simulink model "decoder8to256"  (R2020a)
settings: Solver=VariableStepAuto  StartTime=0.0  StopTime=10.0  RelTol=1e-3
(part 2 of 2)

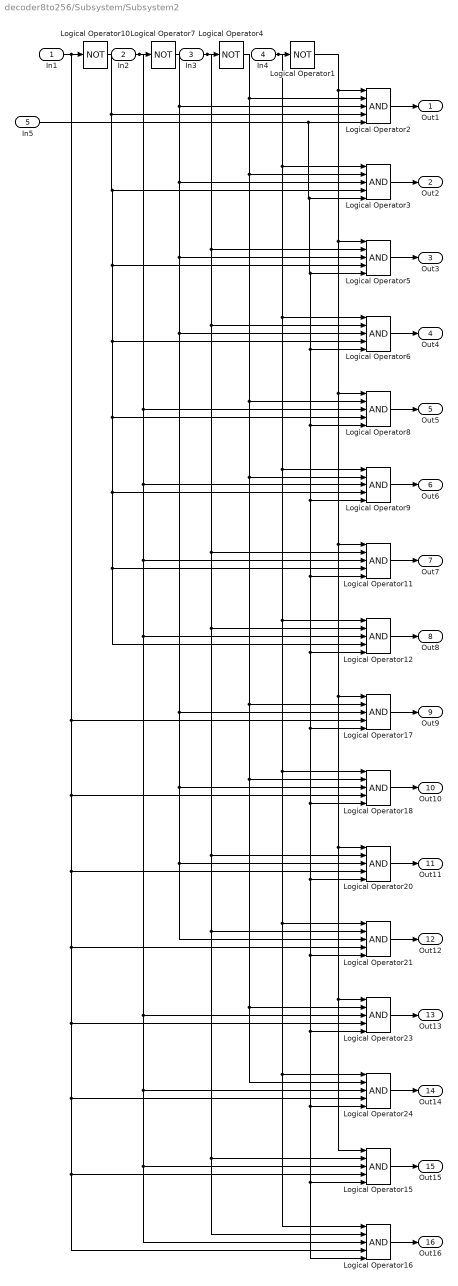
== system decoder8to256/Subsystem/Subsystem2 ==
  In1 : Inport
  In2 : Inport  Port=2
  In3 : Inport  Port=3
  In4 : Inport  Port=4
  In5 : Inport  Port=5
  Logical Operator{1,4,7,10} (4 alike) : Logic  Operator=NOT  AllPortsSameDT=off  OutDataTypeStr=boolean
  Logical Operator{2..3,5..6,8..9,11..12,15..18,20..21,23..24} (16 alike) : Logic  Inputs=5  AllPortsSameDT=off  OutDataTypeStr=boolean
  Out1 : Outport
  Out2 : Outport  Port=2
  Out3 : Outport  Port=3
  Out4 : Outport  Port=4
  Out5 : Outport  Port=5
  Out6 : Outport  Port=6
  Out7 : Outport  Port=7
  Out8 : Outport  Port=8
  Out9 : Outport  Port=9
  Out10 : Outport  Port=10
  Out11 : Outport  Port=11
  Out12 : Outport  Port=12
  Out13 : Outport  Port=13
  Out14 : Outport  Port=14
  Out15 : Outport  Port=15
  Out16 : Outport  Port=16
  wires:
  Logical Operator11/1 -> Out7/1
  Logical Operator12/1 -> Out8/1
  Logical Operator18/1 -> Out10/1
  In2/1 -> Logical Operator16/3, Logical Operator15/3, Logical Operator24/3, Logical Operator23/3, Logical Operator12/3, Logical Operator11/3, Logical Operator9/3, Logical Operator8/3, Logical Operator7/1
  In3/1 -> Logical Operator11/2, Logical Operator15/2, Logical Operator16/2, Logical Operator21/2, Logical Operator20/2, Logical Operator12/2, Logical Operator6/2, Logical Operator5/2, Logical Operator4/1
  Logical Operator24/1 -> Out14/1
  In4/1 -> Logical Operator16/1, Logical Operator24/1, Logical Operator21/1, Logical Operator18/1, Logical Operator12/1, Logical Operator9/1, Logical Operator6/1, Logical Operator3/1, Logical Operator1/1
  Logical Operator10/1 -> Logical Operator12/4, Logical Operator11/4, Logical Operator9/4, Logical Operator8/4, Logical Operator6/4, Logical Operator5/4, Logical Operator3/4, Logical Operator2/4
  Logical Operator9/1 -> Out6/1
  In5/1 -> Logical Operator16/5, Logical Operator15/5, Logical Operator24/5, Logical Operator23/5, Logical Operator21/5, Logical Operator20/5, Logical Operator18/5, Logical Operator17/5, Logical Operator12/5, Logical Operator11/5, Logical Operator9/5, Logical Operator8/5, Logical Operator6/5, Logical Operator5/5, Logical Operator3/5, Logical Operator2/5
  Logical Operator5/1 -> Out3/1
  Logical Operator1/1 -> Logical Operator15/1, Logical Operator23/1, Logical Operator20/1, Logical Operator17/1, Logical Operator11/1, Logical Operator8/1, Logical Operator5/1, Logical Operator2/1
  Logical Operator2/1 -> Out1/1
  Logical Operator21/1 -> Out12/1
  Logical Operator8/1 -> Out5/1
  Logical Operator7/1 -> Logical Operator21/3, Logical Operator20/3, Logical Operator18/3, Logical Operator17/3, Logical Operator6/3, Logical Operator5/3, Logical Operator3/3, Logical Operator2/3
  Logical Operator16/1 -> Out16/1
  Logical Operator15/1 -> Out15/1
  In1/1 -> Logical Operator17/4, Logical Operator18/4, Logical Operator20/4, Logical Operator21/4, Logical Operator23/4, Logical Operator24/4, Logical Operator15/4, Logical Operator16/4, Logical Operator10/1
  Logical Operator3/1 -> Out2/1
  Logical Operator20/1 -> Out11/1
  Logical Operator6/1 -> Out4/1
  Logical Operator23/1 -> Out13/1
  Logical Operator4/1 -> Logical Operator24/2, Logical Operator23/2, Logical Operator18/2, Logical Operator17/2, Logical Operator9/2, Logical Operator8/2, Logical Operator3/2, Logical Operator2/2
  Logical Operator17/1 -> Out9/1

== system decoder8to256/Subsystem/Subsystem3 ==
  In1 : Inport
  In2 : Inport  Port=2
  In3 : Inport  Port=3
  In4 : Inport  Port=4
  In5 : Inport  Port=5
  Logical Operator{1,4,7,10} (4 alike) : Logic  Operator=NOT  AllPortsSameDT=off  OutDataTypeStr=boolean
  Logical Operator{2..3,5..6,8..9,11..12,15..18,20..21,23..24} (16 alike) : Logic  Inputs=5  AllPortsSameDT=off  OutDataTypeStr=boolean
  Out1 : Outport
  Out2 : Outport  Port=2
  Out3 : Outport  Port=3
  Out4 : Outport  Port=4
  Out5 : Outport  Port=5
  Out6 : Outport  Port=6
  Out7 : Outport  Port=7
  Out8 : Outport  Port=8
  Out9 : Outport  Port=9
  Out10 : Outport  Port=10
  Out11 : Outport  Port=11
  Out12 : Outport  Port=12
  Out13 : Outport  Port=13
  Out14 : Outport  Port=14
  Out15 : Outport  Port=15
  Out16 : Outport  Port=16
  wires:
  Logical Operator11/1 -> Out7/1
  Logical Operator12/1 -> Out8/1
  Logical Operator18/1 -> Out10/1
  In2/1 -> Logical Operator16/3, Logical Operator15/3, Logical Operator24/3, Logical Operator23/3, Logical Operator12/3, Logical Operator11/3, Logical Operator9/3, Logical Operator8/3, Logical Operator7/1
  In3/1 -> Logical Operator11/2, Logical Operator15/2, Logical Operator16/2, Logical Operator21/2, Logical Operator20/2, Logical Operator12/2, Logical Operator6/2, Logical Operator5/2, Logical Operator4/1
  Logical Operator24/1 -> Out14/1
  In4/1 -> Logical Operator16/1, Logical Operator24/1, Logical Operator21/1, Logical Operator18/1, Logical Operator12/1, Logical Operator9/1, Logical Operator6/1, Logical Operator3/1, Logical Operator1/1
  Logical Operator10/1 -> Logical Operator12/4, Logical Operator11/4, Logical Operator9/4, Logical Operator8/4, Logical Operator6/4, Logical Operator5/4, Logical Operator3/4, Logical Operator2/4
  Logical Operator9/1 -> Out6/1
  In5/1 -> Logical Operator16/5, Logical Operator15/5, Logical Operator24/5, Logical Operator23/5, Logical Operator21/5, Logical Operator20/5, Logical Operator18/5, Logical Operator17/5, Logical Operator12/5, Logical Operator11/5, Logical Operator9/5, Logical Operator8/5, Logical Operator6/5, Logical Operator5/5, Logical Operator3/5, Logical Operator2/5
  Logical Operator5/1 -> Out3/1
  Logical Operator1/1 -> Logical Operator15/1, Logical Operator23/1, Logical Operator20/1, Logical Operator17/1, Logical Operator11/1, Logical Operator8/1, Logical Operator5/1, Logical Operator2/1
  Logical Operator2/1 -> Out1/1
  Logical Operator21/1 -> Out12/1
  Logical Operator8/1 -> Out5/1
  Logical Operator7/1 -> Logical Operator21/3, Logical Operator20/3, Logical Operator18/3, Logical Operator17/3, Logical Operator6/3, Logical Operator5/3, Logical Operator3/3, Logical Operator2/3
  Logical Operator16/1 -> Out16/1
  Logical Operator15/1 -> Out15/1
  In1/1 -> Logical Operator17/4, Logical Operator18/4, Logical Operator20/4, Logical Operator21/4, Logical Operator23/4, Logical Operator24/4, Logical Operator15/4, Logical Operator16/4, Logical Operator10/1
  Logical Operator3/1 -> Out2/1
  Logical Operator20/1 -> Out11/1
  Logical Operator6/1 -> Out4/1
  Logical Operator23/1 -> Out13/1
  Logical Operator4/1 -> Logical Operator24/2, Logical Operator23/2, Logical Operator18/2, Logical Operator17/2, Logical Operator9/2, Logical Operator8/2, Logical Operator3/2, Logical Operator2/2
  Logical Operator17/1 -> Out9/1

== system decoder8to256/Subsystem/Subsystem4 ==
  In1 : Inport
  In2 : Inport  Port=2
  In3 : Inport  Port=3
  In4 : Inport  Port=4
  In5 : Inport  Port=5
  Logical Operator{1,4,7,10} (4 alike) : Logic  Operator=NOT  AllPortsSameDT=off  OutDataTypeStr=boolean
  Logical Operator{2..3,5..6,8..9,11..12,15..18,20..21,23..24} (16 alike) : Logic  Inputs=5  AllPortsSameDT=off  OutDataTypeStr=boolean
  Out1 : Outport
  Out2 : Outport  Port=2
  Out3 : Outport  Port=3
  Out4 : Outport  Port=4
  Out5 : Outport  Port=5
  Out6 : Outport  Port=6
  Out7 : Outport  Port=7
  Out8 : Outport  Port=8
  Out9 : Outport  Port=9
  Out10 : Outport  Port=10
  Out11 : Outport  Port=11
  Out12 : Outport  Port=12
  Out13 : Outport  Port=13
  Out14 : Outport  Port=14
  Out15 : Outport  Port=15
  Out16 : Outport  Port=16
  wires:
  Logical Operator11/1 -> Out7/1
  Logical Operator12/1 -> Out8/1
  Logical Operator18/1 -> Out10/1
  In2/1 -> Logical Operator16/3, Logical Operator15/3, Logical Operator24/3, Logical Operator23/3, Logical Operator12/3, Logical Operator11/3, Logical Operator9/3, Logical Operator8/3, Logical Operator7/1
  In3/1 -> Logical Operator11/2, Logical Operator15/2, Logical Operator16/2, Logical Operator21/2, Logical Operator20/2, Logical Operator12/2, Logical Operator6/2, Logical Operator5/2, Logical Operator4/1
  Logical Operator24/1 -> Out14/1
  In4/1 -> Logical Operator16/1, Logical Operator24/1, Logical Operator21/1, Logical Operator18/1, Logical Operator12/1, Logical Operator9/1, Logical Operator6/1, Logical Operator3/1, Logical Operator1/1
  Logical Operator10/1 -> Logical Operator12/4, Logical Operator11/4, Logical Operator9/4, Logical Operator8/4, Logical Operator6/4, Logical Operator5/4, Logical Operator3/4, Logical Operator2/4
  Logical Operator9/1 -> Out6/1
  In5/1 -> Logical Operator16/5, Logical Operator15/5, Logical Operator24/5, Logical Operator23/5, Logical Operator21/5, Logical Operator20/5, Logical Operator18/5, Logical Operator17/5, Logical Operator12/5, Logical Operator11/5, Logical Operator9/5, Logical Operator8/5, Logical Operator6/5, Logical Operator5/5, Logical Operator3/5, Logical Operator2/5
  Logical Operator5/1 -> Out3/1
  Logical Operator1/1 -> Logical Operator15/1, Logical Operator23/1, Logical Operator20/1, Logical Operator17/1, Logical Operator11/1, Logical Operator8/1, Logical Operator5/1, Logical Operator2/1
  Logical Operator2/1 -> Out1/1
  Logical Operator21/1 -> Out12/1
  Logical Operator8/1 -> Out5/1
  Logical Operator7/1 -> Logical Operator21/3, Logical Operator20/3, Logical Operator18/3, Logical Operator17/3, Logical Operator6/3, Logical Operator5/3, Logical Operator3/3, Logical Operator2/3
  Logical Operator16/1 -> Out16/1
  Logical Operator15/1 -> Out15/1
  In1/1 -> Logical Operator17/4, Logical Operator18/4, Logical Operator20/4, Logical Operator21/4, Logical Operator23/4, Logical Operator24/4, Logical Operator15/4, Logical Operator16/4, Logical Operator10/1
  Logical Operator3/1 -> Out2/1
  Logical Operator20/1 -> Out11/1
  Logical Operator6/1 -> Out4/1
  Logical Operator23/1 -> Out13/1
  Logical Operator4/1 -> Logical Operator24/2, Logical Operator23/2, Logical Operator18/2, Logical Operator17/2, Logical Operator9/2, Logical Operator8/2, Logical Operator3/2, Logical Operator2/2
  Logical Operator17/1 -> Out9/1

== system decoder8to256/Subsystem/Subsystem5 ==
  In1 : Inport
  In2 : Inport  Port=2
  In3 : Inport  Port=3
  In4 : Inport  Port=4
  In5 : Inport  Port=5
  Logical Operator{1,4,7,10} (4 alike) : Logic  Operator=NOT  AllPortsSameDT=off  OutDataTypeStr=boolean
  Logical Operator{2..3,5..6,8..9,11..12,15..18,20..21,23..24} (16 alike) : Logic  Inputs=5  AllPortsSameDT=off  OutDataTypeStr=boolean
  Out1 : Outport
  Out2 : Outport  Port=2
  Out3 : Outport  Port=3
  Out4 : Outport  Port=4
  Out5 : Outport  Port=5
  Out6 : Outport  Port=6
  Out7 : Outport  Port=7
  Out8 : Outport  Port=8
  Out9 : Outport  Port=9
  Out10 : Outport  Port=10
  Out11 : Outport  Port=11
  Out12 : Outport  Port=12
  Out13 : Outport  Port=13
  Out14 : Outport  Port=14
  Out15 : Outport  Port=15
  Out16 : Outport  Port=16
  wires:
  Logical Operator11/1 -> Out7/1
  Logical Operator12/1 -> Out8/1
  Logical Operator18/1 -> Out10/1
  In2/1 -> Logical Operator16/3, Logical Operator15/3, Logical Operator24/3, Logical Operator23/3, Logical Operator12/3, Logical Operator11/3, Logical Operator9/3, Logical Operator8/3, Logical Operator7/1
  In3/1 -> Logical Operator11/2, Logical Operator15/2, Logical Operator16/2, Logical Operator21/2, Logical Operator20/2, Logical Operator12/2, Logical Operator6/2, Logical Operator5/2, Logical Operator4/1
  Logical Operator24/1 -> Out14/1
  In4/1 -> Logical Operator16/1, Logical Operator24/1, Logical Operator21/1, Logical Operator18/1, Logical Operator12/1, Logical Operator9/1, Logical Operator6/1, Logical Operator3/1, Logical Operator1/1
  Logical Operator10/1 -> Logical Operator12/4, Logical Operator11/4, Logical Operator9/4, Logical Operator8/4, Logical Operator6/4, Logical Operator5/4, Logical Operator3/4, Logical Operator2/4
  Logical Operator9/1 -> Out6/1
  In5/1 -> Logical Operator16/5, Logical Operator15/5, Logical Operator24/5, Logical Operator23/5, Logical Operator21/5, Logical Operator20/5, Logical Operator18/5, Logical Operator17/5, Logical Operator12/5, Logical Operator11/5, Logical Operator9/5, Logical Operator8/5, Logical Operator6/5, Logical Operator5/5, Logical Operator3/5, Logical Operator2/5
  Logical Operator5/1 -> Out3/1
  Logical Operator1/1 -> Logical Operator15/1, Logical Operator23/1, Logical Operator20/1, Logical Operator17/1, Logical Operator11/1, Logical Operator8/1, Logical Operator5/1, Logical Operator2/1
  Logical Operator2/1 -> Out1/1
  Logical Operator21/1 -> Out12/1
  Logical Operator8/1 -> Out5/1
  Logical Operator7/1 -> Logical Operator21/3, Logical Operator20/3, Logical Operator18/3, Logical Operator17/3, Logical Operator6/3, Logical Operator5/3, Logical Operator3/3, Logical Operator2/3
  Logical Operator16/1 -> Out16/1
  Logical Operator15/1 -> Out15/1
  In1/1 -> Logical Operator17/4, Logical Operator18/4, Logical Operator20/4, Logical Operator21/4, Logical Operator23/4, Logical Operator24/4, Logical Operator15/4, Logical Operator16/4, Logical Operator10/1
  Logical Operator3/1 -> Out2/1
  Logical Operator20/1 -> Out11/1
  Logical Operator6/1 -> Out4/1
  Logical Operator23/1 -> Out13/1
  Logical Operator4/1 -> Logical Operator24/2, Logical Operator23/2, Logical Operator18/2, Logical Operator17/2, Logical Operator9/2, Logical Operator8/2, Logical Operator3/2, Logical Operator2/2
  Logical Operator17/1 -> Out9/1

== system decoder8to256/Subsystem/Subsystem6 ==
  In1 : Inport
  In2 : Inport  Port=2
  In3 : Inport  Port=3
  In4 : Inport  Port=4
  In5 : Inport  Port=5
  Logical Operator{1,4,7,10} (4 alike) : Logic  Operator=NOT  AllPortsSameDT=off  OutDataTypeStr=boolean
  Logical Operator{2..3,5..6,8..9,11..12,15..18,20..21,23..24} (16 alike) : Logic  Inputs=5  AllPortsSameDT=off  OutDataTypeStr=boolean
  Out1 : Outport
  Out2 : Outport  Port=2
  Out3 : Outport  Port=3
  Out4 : Outport  Port=4
  Out5 : Outport  Port=5
  Out6 : Outport  Port=6
  Out7 : Outport  Port=7
  Out8 : Outport  Port=8
  Out9 : Outport  Port=9
  Out10 : Outport  Port=10
  Out11 : Outport  Port=11
  Out12 : Outport  Port=12
  Out13 : Outport  Port=13
  Out14 : Outport  Port=14
  Out15 : Outport  Port=15
  Out16 : Outport  Port=16
  wires:
  Logical Operator11/1 -> Out7/1
  Logical Operator12/1 -> Out8/1
  Logical Operator18/1 -> Out10/1
  In2/1 -> Logical Operator16/3, Logical Operator15/3, Logical Operator24/3, Logical Operator23/3, Logical Operator12/3, Logical Operator11/3, Logical Operator9/3, Logical Operator8/3, Logical Operator7/1
  In3/1 -> Logical Operator11/2, Logical Operator15/2, Logical Operator16/2, Logical Operator21/2, Logical Operator20/2, Logical Operator12/2, Logical Operator6/2, Logical Operator5/2, Logical Operator4/1
  Logical Operator24/1 -> Out14/1
  In4/1 -> Logical Operator16/1, Logical Operator24/1, Logical Operator21/1, Logical Operator18/1, Logical Operator12/1, Logical Operator9/1, Logical Operator6/1, Logical Operator3/1, Logical Operator1/1
  Logical Operator10/1 -> Logical Operator12/4, Logical Operator11/4, Logical Operator9/4, Logical Operator8/4, Logical Operator6/4, Logical Operator5/4, Logical Operator3/4, Logical Operator2/4
  Logical Operator9/1 -> Out6/1
  In5/1 -> Logical Operator16/5, Logical Operator15/5, Logical Operator24/5, Logical Operator23/5, Logical Operator21/5, Logical Operator20/5, Logical Operator18/5, Logical Operator17/5, Logical Operator12/5, Logical Operator11/5, Logical Operator9/5, Logical Operator8/5, Logical Operator6/5, Logical Operator5/5, Logical Operator3/5, Logical Operator2/5
  Logical Operator5/1 -> Out3/1
  Logical Operator1/1 -> Logical Operator15/1, Logical Operator23/1, Logical Operator20/1, Logical Operator17/1, Logical Operator11/1, Logical Operator8/1, Logical Operator5/1, Logical Operator2/1
  Logical Operator2/1 -> Out1/1
  Logical Operator21/1 -> Out12/1
  Logical Operator8/1 -> Out5/1
  Logical Operator7/1 -> Logical Operator21/3, Logical Operator20/3, Logical Operator18/3, Logical Operator17/3, Logical Operator6/3, Logical Operator5/3, Logical Operator3/3, Logical Operator2/3
  Logical Operator16/1 -> Out16/1
  Logical Operator15/1 -> Out15/1
  In1/1 -> Logical Operator17/4, Logical Operator18/4, Logical Operator20/4, Logical Operator21/4, Logical Operator23/4, Logical Operator24/4, Logical Operator15/4, Logical Operator16/4, Logical Operator10/1
  Logical Operator3/1 -> Out2/1
  Logical Operator20/1 -> Out11/1
  Logical Operator6/1 -> Out4/1
  Logical Operator23/1 -> Out13/1
  Logical Operator4/1 -> Logical Operator24/2, Logical Operator23/2, Logical Operator18/2, Logical Operator17/2, Logical Operator9/2, Logical Operator8/2, Logical Operator3/2, Logical Operator2/2
  Logical Operator17/1 -> Out9/1

== system decoder8to256/Subsystem/Subsystem7 ==
  In1 : Inport
  In2 : Inport  Port=2
  In3 : Inport  Port=3
  In4 : Inport  Port=4
  In5 : Inport  Port=5
  Logical Operator{1,4,7,10} (4 alike) : Logic  Operator=NOT  AllPortsSameDT=off  OutDataTypeStr=boolean
  Logical Operator{2..3,5..6,8..9,11..12,15..18,20..21,23..24} (16 alike) : Logic  Inputs=5  AllPortsSameDT=off  OutDataTypeStr=boolean
  Out1 : Outport
  Out2 : Outport  Port=2
  Out3 : Outport  Port=3
  Out4 : Outport  Port=4
  Out5 : Outport  Port=5
  Out6 : Outport  Port=6
  Out7 : Outport  Port=7
  Out8 : Outport  Port=8
  Out9 : Outport  Port=9
  Out10 : Outport  Port=10
  Out11 : Outport  Port=11
  Out12 : Outport  Port=12
  Out13 : Outport  Port=13
  Out14 : Outport  Port=14
  Out15 : Outport  Port=15
  Out16 : Outport  Port=16
  wires:
  Logical Operator11/1 -> Out7/1
  Logical Operator12/1 -> Out8/1
  Logical Operator18/1 -> Out10/1
  In2/1 -> Logical Operator16/3, Logical Operator15/3, Logical Operator24/3, Logical Operator23/3, Logical Operator12/3, Logical Operator11/3, Logical Operator9/3, Logical Operator8/3, Logical Operator7/1
  In3/1 -> Logical Operator11/2, Logical Operator15/2, Logical Operator16/2, Logical Operator21/2, Logical Operator20/2, Logical Operator12/2, Logical Operator6/2, Logical Operator5/2, Logical Operator4/1
  Logical Operator24/1 -> Out14/1
  In4/1 -> Logical Operator16/1, Logical Operator24/1, Logical Operator21/1, Logical Operator18/1, Logical Operator12/1, Logical Operator9/1, Logical Operator6/1, Logical Operator3/1, Logical Operator1/1
  Logical Operator10/1 -> Logical Operator12/4, Logical Operator11/4, Logical Operator9/4, Logical Operator8/4, Logical Operator6/4, Logical Operator5/4, Logical Operator3/4, Logical Operator2/4
  Logical Operator9/1 -> Out6/1
  In5/1 -> Logical Operator16/5, Logical Operator15/5, Logical Operator24/5, Logical Operator23/5, Logical Operator21/5, Logical Operator20/5, Logical Operator18/5, Logical Operator17/5, Logical Operator12/5, Logical Operator11/5, Logical Operator9/5, Logical Operator8/5, Logical Operator6/5, Logical Operator5/5, Logical Operator3/5, Logical Operator2/5
  Logical Operator5/1 -> Out3/1
  Logical Operator1/1 -> Logical Operator15/1, Logical Operator23/1, Logical Operator20/1, Logical Operator17/1, Logical Operator11/1, Logical Operator8/1, Logical Operator5/1, Logical Operator2/1
  Logical Operator2/1 -> Out1/1
  Logical Operator21/1 -> Out12/1
  Logical Operator8/1 -> Out5/1
  Logical Operator7/1 -> Logical Operator21/3, Logical Operator20/3, Logical Operator18/3, Logical Operator17/3, Logical Operator6/3, Logical Operator5/3, Logical Operator3/3, Logical Operator2/3
  Logical Operator16/1 -> Out16/1
  Logical Operator15/1 -> Out15/1
  In1/1 -> Logical Operator17/4, Logical Operator18/4, Logical Operator20/4, Logical Operator21/4, Logical Operator23/4, Logical Operator24/4, Logical Operator15/4, Logical Operator16/4, Logical Operator10/1
  Logical Operator3/1 -> Out2/1
  Logical Operator20/1 -> Out11/1
  Logical Operator6/1 -> Out4/1
  Logical Operator23/1 -> Out13/1
  Logical Operator4/1 -> Logical Operator24/2, Logical Operator23/2, Logical Operator18/2, Logical Operator17/2, Logical Operator9/2, Logical Operator8/2, Logical Operator3/2, Logical Operator2/2
  Logical Operator17/1 -> Out9/1

== system decoder8to256/Subsystem/Subsystem8 ==
  In1 : Inport
  In2 : Inport  Port=2
  In3 : Inport  Port=3
  In4 : Inport  Port=4
  In5 : Inport  Port=5
  Logical Operator{1,4,7,10} (4 alike) : Logic  Operator=NOT  AllPortsSameDT=off  OutDataTypeStr=boolean
  Logical Operator{2..3,5..6,8..9,11..12,15..18,20..21,23..24} (16 alike) : Logic  Inputs=5  AllPortsSameDT=off  OutDataTypeStr=boolean
  Out1 : Outport
  Out2 : Outport  Port=2
  Out3 : Outport  Port=3
  Out4 : Outport  Port=4
  Out5 : Outport  Port=5
  Out6 : Outport  Port=6
  Out7 : Outport  Port=7
  Out8 : Outport  Port=8
  Out9 : Outport  Port=9
  Out10 : Outport  Port=10
  Out11 : Outport  Port=11
  Out12 : Outport  Port=12
  Out13 : Outport  Port=13
  Out14 : Outport  Port=14
  Out15 : Outport  Port=15
  Out16 : Outport  Port=16
  wires:
  Logical Operator11/1 -> Out7/1
  Logical Operator12/1 -> Out8/1
  Logical Operator18/1 -> Out10/1
  In2/1 -> Logical Operator16/3, Logical Operator15/3, Logical Operator24/3, Logical Operator23/3, Logical Operator12/3, Logical Operator11/3, Logical Operator9/3, Logical Operator8/3, Logical Operator7/1
  In3/1 -> Logical Operator11/2, Logical Operator15/2, Logical Operator16/2, Logical Operator21/2, Logical Operator20/2, Logical Operator12/2, Logical Operator6/2, Logical Operator5/2, Logical Operator4/1
  Logical Operator24/1 -> Out14/1
  In4/1 -> Logical Operator16/1, Logical Operator24/1, Logical Operator21/1, Logical Operator18/1, Logical Operator12/1, Logical Operator9/1, Logical Operator6/1, Logical Operator3/1, Logical Operator1/1
  Logical Operator10/1 -> Logical Operator12/4, Logical Operator11/4, Logical Operator9/4, Logical Operator8/4, Logical Operator6/4, Logical Operator5/4, Logical Operator3/4, Logical Operator2/4
  Logical Operator9/1 -> Out6/1
  In5/1 -> Logical Operator16/5, Logical Operator15/5, Logical Operator24/5, Logical Operator23/5, Logical Operator21/5, Logical Operator20/5, Logical Operator18/5, Logical Operator17/5, Logical Operator12/5, Logical Operator11/5, Logical Operator9/5, Logical Operator8/5, Logical Operator6/5, Logical Operator5/5, Logical Operator3/5, Logical Operator2/5
  Logical Operator5/1 -> Out3/1
  Logical Operator1/1 -> Logical Operator15/1, Logical Operator23/1, Logical Operator20/1, Logical Operator17/1, Logical Operator11/1, Logical Operator8/1, Logical Operator5/1, Logical Operator2/1
  Logical Operator2/1 -> Out1/1
  Logical Operator21/1 -> Out12/1
  Logical Operator8/1 -> Out5/1
  Logical Operator7/1 -> Logical Operator21/3, Logical Operator20/3, Logical Operator18/3, Logical Operator17/3, Logical Operator6/3, Logical Operator5/3, Logical Operator3/3, Logical Operator2/3
  Logical Operator16/1 -> Out16/1
  Logical Operator15/1 -> Out15/1
  In1/1 -> Logical Operator17/4, Logical Operator18/4, Logical Operator20/4, Logical Operator21/4, Logical Operator23/4, Logical Operator24/4, Logical Operator15/4, Logical Operator16/4, Logical Operator10/1
  Logical Operator3/1 -> Out2/1
  Logical Operator20/1 -> Out11/1
  Logical Operator6/1 -> Out4/1
  Logical Operator23/1 -> Out13/1
  Logical Operator4/1 -> Logical Operator24/2, Logical Operator23/2, Logical Operator18/2, Logical Operator17/2, Logical Operator9/2, Logical Operator8/2, Logical Operator3/2, Logical Operator2/2
  Logical Operator17/1 -> Out9/1

== system decoder8to256/Subsystem/Subsystem9 ==
  In1 : Inport
  In2 : Inport  Port=2
  In3 : Inport  Port=3
  In4 : Inport  Port=4
  In5 : Inport  Port=5
  Logical Operator{1,4,7,10} (4 alike) : Logic  Operator=NOT  AllPortsSameDT=off  OutDataTypeStr=boolean
  Logical Operator{2..3,5..6,8..9,11..12,15..18,20..21,23..24} (16 alike) : Logic  Inputs=5  AllPortsSameDT=off  OutDataTypeStr=boolean
  Out1 : Outport
  Out2 : Outport  Port=2
  Out3 : Outport  Port=3
  Out4 : Outport  Port=4
  Out5 : Outport  Port=5
  Out6 : Outport  Port=6
  Out7 : Outport  Port=7
  Out8 : Outport  Port=8
  Out9 : Outport  Port=9
  Out10 : Outport  Port=10
  Out11 : Outport  Port=11
  Out12 : Outport  Port=12
  Out13 : Outport  Port=13
  Out14 : Outport  Port=14
  Out15 : Outport  Port=15
  Out16 : Outport  Port=16
  wires:
  Logical Operator11/1 -> Out7/1
  Logical Operator12/1 -> Out8/1
  Logical Operator18/1 -> Out10/1
  In2/1 -> Logical Operator16/3, Logical Operator15/3, Logical Operator24/3, Logical Operator23/3, Logical Operator12/3, Logical Operator11/3, Logical Operator9/3, Logical Operator8/3, Logical Operator7/1
  In3/1 -> Logical Operator11/2, Logical Operator15/2, Logical Operator16/2, Logical Operator21/2, Logical Operator20/2, Logical Operator12/2, Logical Operator6/2, Logical Operator5/2, Logical Operator4/1
  Logical Operator24/1 -> Out14/1
  In4/1 -> Logical Operator16/1, Logical Operator24/1, Logical Operator21/1, Logical Operator18/1, Logical Operator12/1, Logical Operator9/1, Logical Operator6/1, Logical Operator3/1, Logical Operator1/1
  Logical Operator10/1 -> Logical Operator12/4, Logical Operator11/4, Logical Operator9/4, Logical Operator8/4, Logical Operator6/4, Logical Operator5/4, Logical Operator3/4, Logical Operator2/4
  Logical Operator9/1 -> Out6/1
  In5/1 -> Logical Operator16/5, Logical Operator15/5, Logical Operator24/5, Logical Operator23/5, Logical Operator21/5, Logical Operator20/5, Logical Operator18/5, Logical Operator17/5, Logical Operator12/5, Logical Operator11/5, Logical Operator9/5, Logical Operator8/5, Logical Operator6/5, Logical Operator5/5, Logical Operator3/5, Logical Operator2/5
  Logical Operator5/1 -> Out3/1
  Logical Operator1/1 -> Logical Operator15/1, Logical Operator23/1, Logical Operator20/1, Logical Operator17/1, Logical Operator11/1, Logical Operator8/1, Logical Operator5/1, Logical Operator2/1
  Logical Operator2/1 -> Out1/1
  Logical Operator21/1 -> Out12/1
  Logical Operator8/1 -> Out5/1
  Logical Operator7/1 -> Logical Operator21/3, Logical Operator20/3, Logical Operator18/3, Logical Operator17/3, Logical Operator6/3, Logical Operator5/3, Logical Operator3/3, Logical Operator2/3
  Logical Operator16/1 -> Out16/1
  Logical Operator15/1 -> Out15/1
  In1/1 -> Logical Operator17/4, Logical Operator18/4, Logical Operator20/4, Logical Operator21/4, Logical Operator23/4, Logical Operator24/4, Logical Operator15/4, Logical Operator16/4, Logical Operator10/1
  Logical Operator3/1 -> Out2/1
  Logical Operator20/1 -> Out11/1
  Logical Operator6/1 -> Out4/1
  Logical Operator23/1 -> Out13/1
  Logical Operator4/1 -> Logical Operator24/2, Logical Operator23/2, Logical Operator18/2, Logical Operator17/2, Logical Operator9/2, Logical Operator8/2, Logical Operator3/2, Logical Operator2/2
  Logical Operator17/1 -> Out9/1
